simulink model "pwm_mod_demod"  (R2020a)
settings: Solver=VariableStepAuto  StartTime=0.0  StopTime=10.0  RelTol=1e-3
libraries: dsparch4 x2, commutil2 x2, commsrccod2 x2
settings Model: Creator=91735  LastModifiedBy=91735

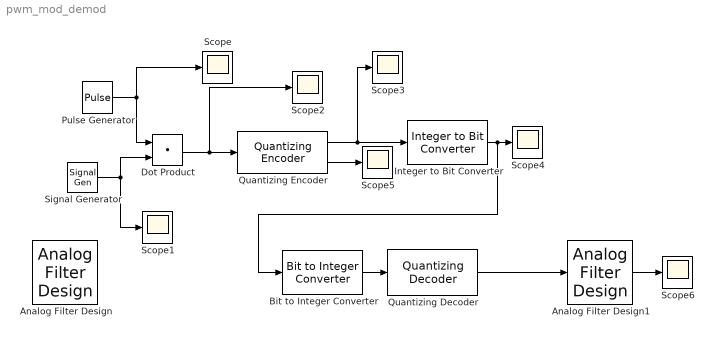
== system pwm_mod_demod ==
  Analog Filter Design : dsparch4/Analog Filter Design  method=Butterworth  filttype=Lowpass  N=8  Wlo=30  Whi=80  Rp=2  Rs=40
  Analog Filter Design1 : dsparch4/Analog Filter Design  method=Butterworth  filttype=Lowpass  N=8  Wlo=30  Whi=80  Rp=2  Rs=40
  Bit to Integer Converter : commutil2/Bit to Integer Converter  nbits=4  bitOrder=MSB first  signedOutputValues=Unsigned  outDtype=Inherit via internal rule  outDtypeSigned=Inherit via internal rule
  Dot Product : DotProduct  InputSameDT=on  OutDataTypeStr=Inherit: Inherit via internal rule
  Integer to Bit Converter : commutil2/Integer to Bit Converter  nbits=4  signedInputValues=Unsigned  bitOrder=MSB first  outDtype=Inherit via internal rule
  Pulse Generator : DiscretePulseGenerator  PulseType=Time based  Period=0.01
  Quantizing Decoder : commsrccod2/Quantizing Decoder  codebook=[-.5 0 0.5]  QuDType=double
      settings: SourceProductBaseCode=CM
  Quantizing Encoder : commsrccod2/Quantizing Encoder  partition=[-.5 0 0.5]  codebook=[-0.75 -0.25 0.25 0.75]  idxDType=double
      settings: SourceProductBaseCode=CM
  Scope{,1..6} (7 alike) : Scope
  Signal Generator : SignalGenerator  Amplitude=2  Frequency=5  Units=rad/sec
  wires:
  Signal Generator/1 -> Scope1/1, Dot Product/2
  Pulse Generator/1 -> Scope/1, Dot Product/1
  Dot Product/1 -> Scope2/1, Quantizing Encoder/1
  Quantizing Encoder/1 -> Scope3/1, Integer to Bit Converter/1
  Integer to Bit Converter/1 -> Bit to Integer Converter/1, Scope4/1
  Quantizing Encoder/2 -> Scope5/1
  Bit to Integer Converter/1 -> Quantizing Decoder/1
  Quantizing Decoder/1 -> Analog Filter Design1/1
  Analog Filter Design1/1 -> Scope6/1
